simulink model "Pos_CBAgent"  (Simulink 7.1)
settings: Solver=ode45  SolverMode=SingleTasking  StartTime=0.0  StopTime=10.0  RelTol=1e-3  AbsTol=1e-6
settings Model: Creator=The MathWorks Inc.  LastModifiedBy=suarezjl  ExtModeTrigMode=oneshot  ExtModeArmWhenConnect=off  ExtModeAutoUpdateStatusClock=off
settings DataIOCC: LimitDataPoints=off  SignalLoggingName=logsOut
settings OptimizationCC: BooleanDataType=off  InlineInvariantSignals=on
settings DebuggingCC: SaveWithParameterizedLinksMsg=none  CheckExecutionContextPreStartOutputMsg=on  CheckExecutionContextRuntimeOutputMsg=on  SignalResolutionControl=TryResolveAllWithWarning  SolverPrmCheckMsg=none  MultiTaskDSMMsg=warning  MultiTaskCondExecSysMsg=none  IntegerOverflowMsg=none  StrictBusMsg=None
settings HardwareCC: TargetUnknown=on
settings ModelReferenceCC: UpdateModelReferenceTargets=IfOutOfDate
settings RTWCC: IncludeERTFirstTime=on
settings GRTTargetCC: TargetFcnLib=ansi_tfl_tmw.mat

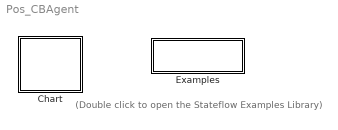
== system Pos_CBAgent ==
  note: (Double click to open the
      | Stateflow Examples Library)
  Chart : Stateflow chart
  Examples : Subsystem
      settings: OpenFcn=sf('Private','sf_examples')
      mask Display: disp('Examples')

== system Pos_CBAgent/Examples ==

== stateflow chart Chart ==
  state Initialize
    \\Octavia\ISACControlBasisModule\RightModule\Arm\ArmController.DoHomingRoutine()
    \\Octavia\ISACControlBasisModule\IKinCB\StateMachine.Wait(5000)
    \\Octavia\ISACControlBasisModule\LeftModule\Arm\ArmController.DoHomingRoutine()
    \\Octavia\ISACControlBasisModule\IKinCB\StateMachine.Wait(5000)
    \\Octavia\ISACControlBasisModule\IKinCB\IKinLeft.Initialize()
    \\Octavia\ISACControlBasisModule\IKinCB\IKinRight.Initialize()
    \\Octavia\ISACControlBasisModule\IKinCB\FKinLeft.Initialize()
    \\Octavia\ISACControlBasisModule\IKinCB\FKinRight.Initialize()
    \\Octavia\ISACControlBasisModule\IKinCB\IKinCBLeft.Initialize()
    \\Octavia\ISACControlBasisModule\IKinCB\IKinCBRight.Initialize()
  state ControlBasis
    \\Octavia\ISACControlBasisModule\LeftModule\Arm\ArmController.Move()
    \\Octavia\ISACControlBasisModule\RightModule\Arm\ArmController.Move()
    \\Octavia\ISACControlBasisModule\IKinCB\FKinLeft.kin_ForwardKinematics()
    \\Octavia\ISACControlBasisModule\IKinCB\FKinRight.kin_ForwardKinematics()
    \\Octavia\ISACControlBasisModule\IKinCB\IKinCBLeft.ComputeControlBasis()
    \\Octavia\ISACControlBasisModule\IKinCB\IKinCBRight.ComputeControlBasis()
    \\Octavia\ISACControlBasisModule\IKinCB\IKinLeft.kin_InverseKinematics()
    \\Octavia\ISACControlBasisModule\IKinCB\IKinRight.kin_InverseKinematics()
  state End
    \\Octavia\ISACControlBasisModule\IKinCB\IKinCBLeft.Close()
    \\Octavia\ISACControlBasisModule\IKinCB\IKinCBRight.Close()
  (default) -> Initialize : Start
  Initialize -> ControlBasis : Signal="Next"
  ControlBasis -> ControlBasis [order 1] : Default
  ControlBasis -> End [order 2] : Signal="Next"
